simulink model "task3"  (R2023b)
settings: Solver=FixedStepDiscrete  StartTime=0.0  StopTime=(12+4)*8-1  RelTol=1e-3
libraries: dspsigops x2, commchan3 x1, dspsrcs4 x1
settings Model: LastModifiedBy=AMEY THAKUR
settings OptimizationCC: ReuseModelBlockBuffer=off

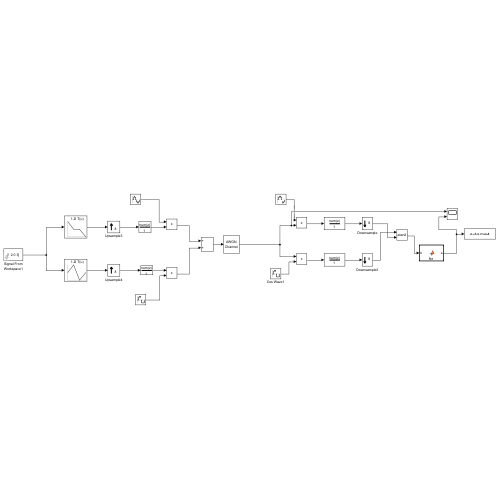
[thumbnail: Simulink's stored preview of the top-level diagram]
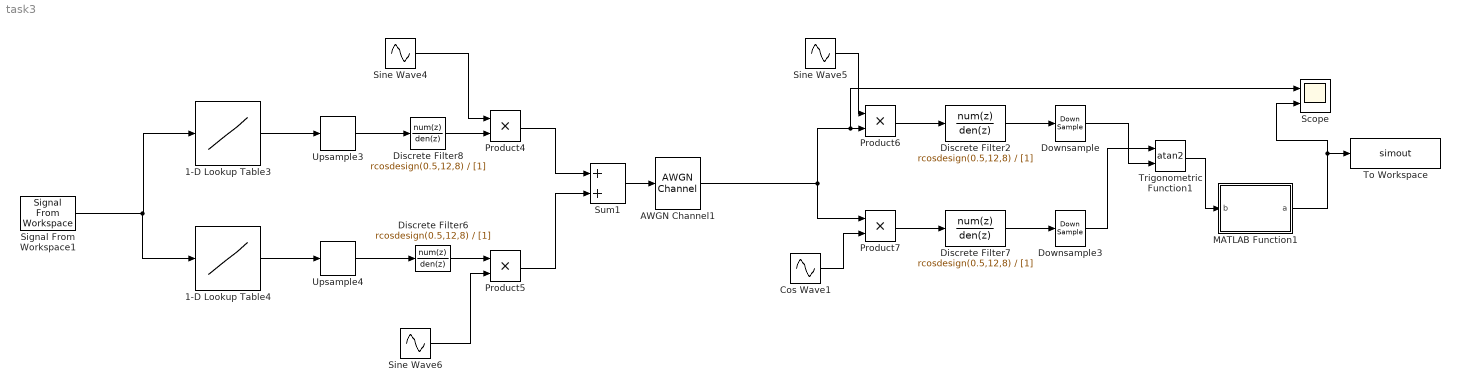
== system task3 ==
  1-D Lookup Table3 : Lookup_n-D  NumberOfTableDimensions=1  BreakpointsForDimension1=[0 1 2 3]  Table=[3 0 0 -3]  InternalRulePriority=Speed  RndMeth=Simplest
  1-D Lookup Table4 : Lookup_n-D  NumberOfTableDimensions=1  BreakpointsForDimension1=[0 1 2 3]  Table=[0 3 -3 0]  InternalRulePriority=Speed  RndMeth=Simplest
  AWGN Channel1 : commchan3/AWGN Channel  LegacyMode=off  NoiseMethod="Signal to noise ratio  (Es/No)"  noiseMode="Signal to noise ratio  (SNR)"  EbNo=10  EsNo=40  SNR=10  BitsPerSymbol=1  SignalPower=1  SamplesPerSymbol=1  SymbolPeriod=1  VarianceSource=Parameter  Variance=1  RandomStream=mt19937ar with seed  Seed=110107589  SimulateUsing=Code generation
  Cos Wave1 : Sin  Amplitude=-sqrt(2)  Frequency=0.5*pi  SampleTime=1
  Discrete Filter{2,6..8} (4 alike) : DiscreteFilter  Numerator=rcosdesign(0.5,12,8)  Denominator=[1]
  Downsample : DownSample  N=8  RateOptions=Allow multirate processing
  Downsample3 : DownSample  N=8  RateOptions=Allow multirate processing
  MATLAB Function1 : MATLAB Function  TreatAsAtomicUnit=on
  Product{4..7} (4 alike) : Product
  Scope : Scope  NumInputPorts=2
  Signal From Workspace1 : dspsrcs4/Signal From Workspace  X=[1 2 0 3]  Ts=8  nsamps=1  OutputAfterFinalValue=Setting to zero  ignoreOrWarnInputAndFrameLengths=off  OutputFrames=off
  Sine Wave4 : Sin  Amplitude=sqrt(2)  Frequency=0.5*pi  Phase=pi/2  SampleTime=1
  Sine Wave5 : Sin  Amplitude=sqrt(2)  Frequency=0.5*pi  Phase=pi/2  SampleTime=1
  Sine Wave6 : Sin  Amplitude=-sqrt(2)  Frequency=0.5*pi  SampleTime=1
  Sum1 : Sum
  To Workspace : ToWorkspace  VariableName=simout  SaveFormat=Timeseries  SampleTime=-1
  Trigonometric Function1 : Trigonometry  Operator=atan2
  Upsample3 : dspsigops/Upsample  FactorSource=Dialog parameter  N=8  Nmax=16  phase=0  RateOptions=Allow multirate processing  ic=0  mode=Unused parameter value
      settings: LibrarySourceBlock=dsphdlsupportsigops/Upsample
  Upsample4 : dspsigops/Upsample  FactorSource=Dialog parameter  N=8  Nmax=16  phase=0  RateOptions=Allow multirate processing  ic=0  mode=Unused parameter value
      settings: LibrarySourceBlock=dsphdlsupportsigops/Upsample
  wires:
  Downsample3/1 -> Trigonometric Function1/1
  Downsample/1 -> Trigonometric Function1/2
  MATLAB Function1/1(a) -> To Workspace/1, Scope/2
  Discrete Filter2/1 -> Downsample/1
  Product7/1 -> Discrete Filter7/1
  Sine Wave5/1 -> Product6/1
  Discrete Filter7/1 -> Downsample3/1
  Cos Wave1/1 -> Product7/2
  Product6/1 -> Discrete Filter2/1
  Trigonometric Function1/1 -> MATLAB Function1/1(b)
  Sine Wave4/1 -> Product4/1
  1-D Lookup Table3/1 -> Upsample3/1
  Sine Wave6/1 -> Product5/2
  Upsample3/1 -> Discrete Filter8/1
  Signal From Workspace1/1 -> 1-D Lookup Table4/1, 1-D Lookup Table3/1
  Product4/1 -> Sum1/1
  Upsample4/1 -> Discrete Filter6/1
  Discrete Filter8/1 -> Product4/2
  Discrete Filter6/1 -> Product5/1
  Product5/1 -> Sum1/2
  1-D Lookup Table4/1 -> Upsample4/1
  AWGN Channel1/1 -> Product7/1, Scope/1, Product6/2
  Sum1/1 -> AWGN Channel1/1

== matlab function task3/MATLAB Function1 ==
  data: b input; a output
function a = fcn(b)
a=zeros(size(b));
for i=1:length(b)
    if b(i)>=-pi/4 && b(i) < pi/4
        a(i)=0;
    elseif b(i)>=pi/4 && b(i)<3*pi/4
        a(i)=1;
    elseif b(i)>=-3*pi/4 && b(i)<-pi/4
        a(i)=2;
    else
        a(i)=3;
    end
end
